simulink model "Kalman_sim_R2021a"  (R2021a)
settings: Solver=ode1  StartTime=0.0  StopTime=0.03  FixedStep=Ts  RelTol=1e-3
values from neighbouring files (symbols this model uses):
  A = [-R/Ld,         N*Lq*x3_op/Ld,      N*Lq*x2_op/Ld ... (first row only)    [PMSM_Kalman_Filter.m]
  B = [1/Ld, 0 ... (first row only)    [PMSM_Kalman_Filter.m]
  C = eye(3)    [PMSM_Kalman_Filter.m]
  G = eye(3)    [PMSM_Kalman_Filter.m]
  Q = diag(Q_vec)    [PMSM_Kalman_Filter.m]
  Q_vec = ones(3,1)*(w^2)    [PMSM_Kalman_Filter.m]
  R = diag(R_vec)    [PMSM_Kalman_Filter.m]
  R_vec = ones(3,1)*(eta^2)    [PMSM_Kalman_Filter.m]
  Ts = 0.00001    (= 1e-05)    [PMSM_Kalman_Filter.m]
  zero_arr = zeros(3,1)    [PMSM_Kalman_Filter.m]
libraries: aerolibanimutils x1
settings Model: Creator=kiq  LastModifiedBy=kiq
settings DebuggingCC: UnderSpecifiedDimensionMsg=warning

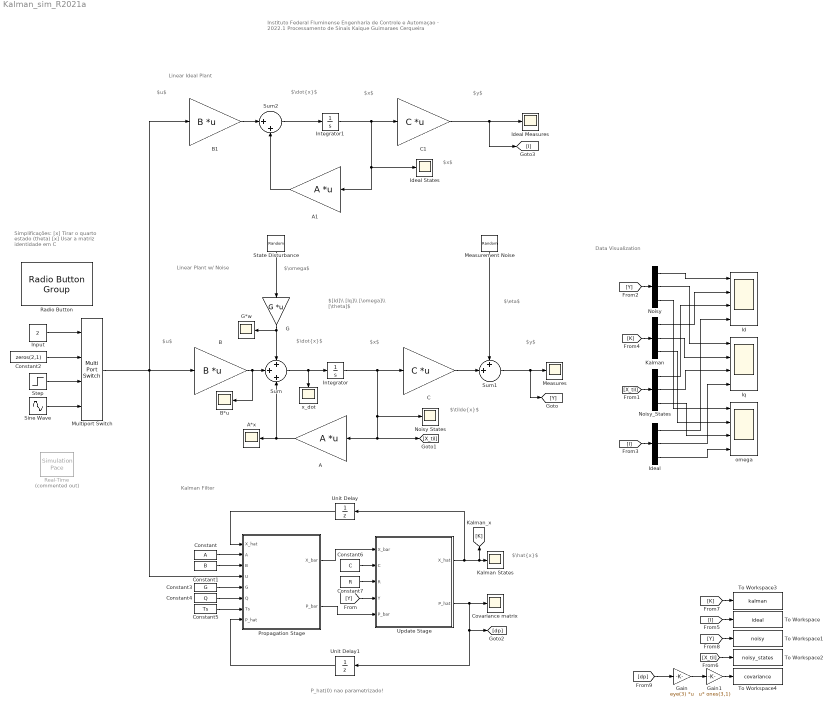
== system Kalman_sim_R2021a ==
  note: Instituto Federal Fluminense
      | Engenharia de Controle e Automaçao - 2022.1
      | Processamento de Sinais
      | Kaique Guimaraes Cerqueira
  note: Data Visualization
  note: P_hat(0) nao parametrizado!
  note: Simplificações:
      | [x] Tirar o quarto estado (theta)
      | [x] Usar a matriz identidade em C
  note: $[Id]\\ [Iq]\\ [\omega]\\ [\theta]$
  note: $\hat{x}$
  note: $x$
  note: Kalman Filter
  note: Linear Plant w/ Noise
  note: $\omega$
  note: $\eta$
  note: $y$
  note: $u$
  note: $x$
  note: $\dot{x}$
  note: $y$
  note: $x$
  note: $u$
  note: $\dot{x}$
  note: Linear Ideal Plant
  note: $\tilde{x}$
  A : Gain  Gain=A  Multiplication=Matrix(K*u)
  A*x : Scope
  A1 : Gain  Gain=A  Multiplication=Matrix(K*u)
  B : Gain  Gain=B  Multiplication=Matrix(K*u)
  B*u : Scope
  B1 : Gain  Gain=B  Multiplication=Matrix(K*u)
  C : Gain  Gain=C  Multiplication=Matrix(K*u)
  C1 : Gain  Gain=C  Multiplication=Matrix(K*u)
  Constant : Constant  Value=A  VectorParams1D=off
  Constant1 : Constant  Value=B  VectorParams1D=off
  Constant2 : Constant  Value=zeros(2,1)  VectorParams1D=off  SampleTime=-1
  Constant3 : Constant  Value=G  VectorParams1D=off
  Constant4 : Constant  Value=Q  VectorParams1D=off
  Constant5 : Constant  Value=Ts  VectorParams1D=off
  Constant6 : Constant  Value=C  VectorParams1D=off
  Constant7 : Constant  Value=R  VectorParams1D=off
  Covariance matrix : Scope
  G : Gain  Gain=G  Multiplication=Matrix(K*u)
  G*w : Scope
  Gain : Gain  Gain=eye(3)  Multiplication=Matrix(K*u)
  Gain1 : Gain  Gain=ones(3,1)  Multiplication=Matrix(u*K)
  Id : Scope  NumInputPorts=4
  Ideal : Demux  Outputs=3
  Ideal Measures : Scope
  Ideal States : Scope
  Input : Constant  Value=2
  Integrator : Integrator
  Integrator1 : Integrator
  Iq : Scope  NumInputPorts=4
  Kalman : Demux  Outputs=3
  Kalman States : Scope
  Measurement Noise : RandomNumber  Mean=zero_arr  Variance=R_vec  Seed=randi(1000,3,1)  VectorParams1D=off
  Measures : Scope
  Multiport Switch : MultiPortSwitch
  Noisy : Demux  Outputs=3
  Noisy States : Scope
  Noisy_States : Demux  Outputs=3
  Propagation Stage : MATLAB Function  TreatAsAtomicUnit=on
  Radio Button : RadioButtonGroup  LabelPosition=Hide  SelectedLabel=Step  ButtonGroupName=Inputs
      settings: Values={{'Zero', 'Step', 'Sine Wave'}, [1 2 3]}
  Real-Time : aerolibanimutils/Simulation Pace  Commented=on  SimulationPace=1  SleepMode=Auto  OutputPaceError=off  SampleTime=-1
  Sine Wave : Sin  Amplitude=[0.001;0.001]  Frequency=2*pi/5  SampleTime=0
  State Disturbance : RandomNumber  Mean=zero_arr  Variance=Q_vec  Seed=randi(1000,3,1)  VectorParams1D=off
  Step : Step  Time=0.001  Before=[0;0]  After=[1;0]  VectorParams1D=off
  Sum : Sum  Inputs=+++
  Sum1 : Sum  Inputs=++|
  Sum2 : Sum  Inputs=|++
  To Workspace : ToWorkspace  VariableName=ideal  SampleTime=-1
  To Workspace1 : ToWorkspace  VariableName=noisy  SampleTime=-1
  To Workspace2 : ToWorkspace  VariableName=noisy_states  SampleTime=-1
  To Workspace3 : ToWorkspace  VariableName=kalman  SampleTime=-1
  To Workspace4 : ToWorkspace  VariableName=covariance  SampleTime=-1
  Unit Delay : UnitDelay  InitialCondition=zero_arr  SampleTime=-1  HasFrameUpgradeWarning=on
  Unit Delay1 : UnitDelay  InitialCondition=eye(3)*999  SampleTime=-1  HasFrameUpgradeWarning=on
  Update Stage : MATLAB Function  TreatAsAtomicUnit=on
  omega : Scope  NumInputPorts=4
  x_dot : Scope
  wires:
  Integrator/1 -> [X_til], A/1, Noisy States/1, C/1
  B/1 -> B*u/1, Sum/2
  A/1 -> Sum/3, A*x/1
  C/1 -> Sum1/2
  Sum1/1 -> [Y], Measures/1
  G/1 -> Sum/1, G*w/1
  Sum/1 -> x_dot/1, Integrator/1
  Input/1 -> Multiport Switch/1
  Constant1/1 -> Propagation Stage/3(B)
  Update Stage/1(X_hat) -> [K], Kalman States/1, Unit Delay/1
  Propagation Stage/1(X_bar) -> Update Stage/1(X_bar)
  Propagation Stage/2(P_bar) -> Update Stage/5(P_bar)
  Constant7/1 -> Update Stage/3(R)
  Constant6/1 -> Update Stage/2(C)
  Constant4/1 -> Propagation Stage/6(Q)
  Constant5/1 -> Propagation Stage/7(Ts)
  Constant3/1 -> Propagation Stage/5(G)
  Constant/1 -> Propagation Stage/2(A)
  Sum2/1 -> Integrator1/1
  Integrator1/1 -> A1/1, Ideal States/1, C1/1
  C1/1 -> [I], Ideal Measures/1
  B1/1 -> Sum2/1
  A1/1 -> Sum2/2
  Unit Delay/1 -> Propagation Stage/1(X_hat)
  Multiport Switch/1 -> B/1, B1/1, Propagation Stage/4(U)
  Constant2/1 -> Multiport Switch/2
  Step/1 -> Multiport Switch/3
  Sine Wave/1 -> Multiport Switch/4
  Update Stage/2(P_hat) -> [dp], Unit Delay1/1, Covariance matrix/1
  [Y] -> Update Stage/4(Y)
  Unit Delay1/1 -> Propagation Stage/8(P_hat)
  [K] -> Kalman/1
  [Y] -> Noisy/1
  [I] -> Ideal/1
  [X_til] -> Noisy_States/1
  Noisy/1 -> Id/1
  Noisy/2 -> Iq/1
  Noisy/3 -> omega/1
  Kalman/1 -> Id/2
  Kalman/2 -> Iq/2
  Kalman/3 -> omega/2
  Noisy_States/1 -> Id/3
  Noisy_States/2 -> Iq/3
  Noisy_States/3 -> omega/3
  Ideal/1 -> Id/4
  Ideal/2 -> Iq/4
  Ideal/3 -> omega/4
  [I] -> To Workspace/1
  [X_til] -> To Workspace2/1
  [K] -> To Workspace3/1
  [Y] -> To Workspace1/1
  [dp] -> Gain/1
  Gain1/1 -> To Workspace4/1
  Gain/1 -> Gain1/1
  State Disturbance/1 -> G/1
  Measurement Noise/1 -> Sum1/1

== matlab function Kalman_sim_R2021a/Propagation Stage ==
  data: X_hat input; A input; X_bar output; B input; U input; G input; Q input; Ts input; P_hat input; P_bar output
function [X_bar, P_bar] = kalman_propagation(X_hat, A, B, U, G, Q, Ts, P_hat)
% Kalman Filter Propagation Stage using Euler1 numerical integration
% 
% ==========================Signals=================================
% X_bar, P_bar -> Estimative based on previous measurements
% X_hat, P_hat -> Estimative based on current measurement (delayed by Z⁻¹)
% A, B, G, Q -> State-space model (w/ noise) matrices
% U -> Input signal (ideal)
% Ts -> Sampling period
%     Compute derivatives
    X_bar_dot = A*X_hat + B*U;
%     P_bar_dot = A*P_hat + P_hat*(A') + G*Q*(G');
    P_bar_dot = A*P_hat + P_hat*transpose(A) + G*Q*transpose(G);
%     Numerical integration
    X_bar = X_bar_dot*Ts + X_hat;
    P_bar = P_bar_dot*Ts + P_hat;
end

== matlab function Kalman_sim_R2021a/Update Stage ==
  data: X_bar input; X_hat output; P_hat output; C input; R input; Y input; P_bar input
function [X_hat, P_hat] = kalman_update(X_bar, C, R, Y, P_bar)
% Kalman Filter Update Stage
% 
% ==========================Signals=================================
% X_hat, P_hat -> Estimative based on current measurement
% X_bar, P_bar -> Estimative based on previous measurements
% C, R -> State-space model (w/ noise) matrices
% Y -> Measurement (sensor) signal corrupted

% Compute Kalman Gain (teoretical result):
%     K = P_bar*(C')*inv(C*P_bar*(C') + R);
    K = P_bar*transpose(C)*inv(C*P_bar*transpose(C) + R);
% -----------------Matlab warning!!!---------------------------------
% Never use the inverse of a matrix to solve a linear system Ax=b with 
% x=inv(A)*b, because it is slow and inaccurate. Suggested Action:
% Instead of multiplying by the inverse, use matrix right division (/) or 
% matrix left division (\). That is:
% -> Replace inv(A)*b with A\b
% -> Replace b*inv(A) with b/A
%     K = P_bar*((C')/(C*P_bar*(C') + R));
    
% Update:
    X_hat = X_bar + K*(Y - C*X_bar);
    P_hat = P_bar - (K*C*P_bar);
end
